simulink model "SpectrumAnalyzerMeasurements"  (R2024a)
settings: Solver=FixedStepDiscrete  StartTime=0.0  StopTime=100  RelTol=1e-3  EnableMultiTasking=on
libraries: dspsrcs4 x10, dsppolyfun x4, dspmlti4 x1
settings Model: Creator=The MathWorks, Inc.  LastModifiedBy=The MathWorks, Inc.
settings SolverCC: AlgebraicLoopSolver=TrustRegion  MaxZcPerStep=1
settings DataIOCC: LimitDataPoints=on  SaveFormat=Array  ReturnWorkspaceOutputs=off
settings OptimizationCC: LifeSpan=inf  SimCompilerOptimization=on
settings DebuggingCC: SolverPrmCheckMsg=warning  UnconnectedInputMsg=warning  UnconnectedOutputMsg=warning  UnconnectedLineMsg=warning  AllowSymbolicDim=off  SymbolicDimsDataTypeCodeGenerationDiagnostic=none  SFUnexpectedBacktrackingDiag=warning  SFNoUnconditionalDefaultTransitionDiag=warning  SFExecutionAtInitializationDiag=none  ArithmeticOperatorsInVariantConditions=warning
settings HardwareCC: ProdBitPerPointer=32  ProdBitPerSizeT=32  ProdBitPerPtrDiffT=32  ProdLargestAtomicFloat=None  ProdIntDivRoundTo=Undefined  ProdEndianess=Unspecified  ProdWordSize=32  ProdHWDeviceType=32-bit Generic
settings ModelReferenceCC: EnableRefExpFcnMdlSchedulingChecks=on  PropagateSignalLabelsOutOfModel=off
settings SFSimCC: SimUseLocalCustomCode=off  SimGenImportedTypeDefs=on  CustomCodeUndefinedFunction=UseInterfaceOnly
settings RTWCC: RTWUseLocalCustomCode=off  GPUComputeCapability=3.5  DLArmComputeVersion=19.05
settings CodeAppCC: StateflowObjectComments=on
settings GRTTargetCC: TargetLangStandard=C89/C90 (ANSI)
settings ConfigComp: CovMetricSettings=dw  CovSaveCumulativeToWorkspaceVar=on  CovSaveSingleToWorkspaceVar=on  CovExternalEMLEnable=off  CovSFcnEnable=off

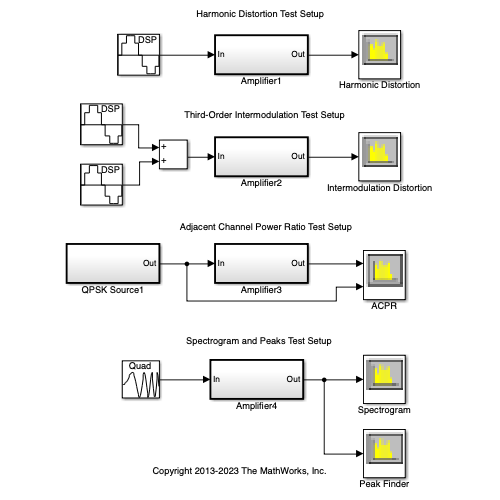
[thumbnail: Simulink's stored preview of the top-level diagram]
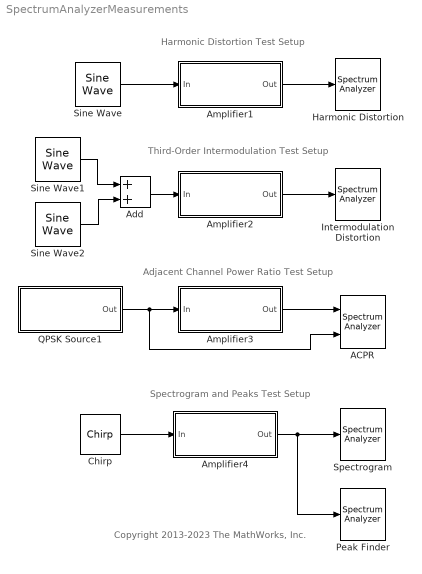
== system SpectrumAnalyzerMeasurements ==
  note: Spectrogram and Peaks Test Setup
  note: Adjacent Channel Power Ratio Test Setup
  note: Third-Order Intermodulation Test Setup
  note: Harmonic Distortion Test Setup
  note: Copyright 2013-2023 The MathWorks, Inc.
  ACPR : SpectrumAnalyzer  NumInputPorts=2  WindowPosition=[162.000000,32.000000,534.000000,420.000000,]  ScopeFrameLocation=window  Method=Welch  SampleRate=38400000  Span=1  StartFrequency=-0.5  StopFrequency=0.5  AveragingMethod=Running  YLabel=dBm  YLimits=[-119.21723774,40.57878414]  ShowLegend=on  AllowFFTLengthLessThanSamplesPerUpdate=on
  Add : Sum
  Amplifier1 : Subsystem  TreatAsAtomicUnit=on
  Amplifier2 : Subsystem  TreatAsAtomicUnit=on
  Amplifier3 : Subsystem  TreatAsAtomicUnit=on
  Amplifier4 : Subsystem  TreatAsAtomicUnit=on
  Chirp : dspsrcs4/Chirp  sweep=Quadratic  mode=Bidirectional  f0=2.5e6  f1=5e6  t1=1e-3  Tsweep=1e-3  phase=0  Ts=1/10/3.84e6  spf=10  datatype=double  OutputFrames=off
  Harmonic Distortion : SpectrumAnalyzer  WindowPosition=[109.000000,45.000000,549.000000,470.000000,]  ScopeFrameLocation=window  Method=Welch  SampleRate=38400000  PlotAsTwoSidedSpectrum=off  RBW=200e3  Span=500  CenterFrequency=250  StartFrequency=0  StopFrequency=500  Window=Kaiser  SidelobeAttenuation=190  OverlapPercent=80  AveragingMethod=Running  YLabel=dBm  YLimits=[-219.95441853,53.99786682]  SelectedToolstripTab=spectrumAnalyzerToolstrip.measurementsTab  AllowFFTLengthLessThanSamplesPerUpdate=on
  Intermodulation Distortion : SpectrumAnalyzer  WindowPosition=[136.000000,50.000000,548.000000,434.000000,]  ScopeFrameLocation=window  Method=Welch  SampleRate=38400000  PlotAsTwoSidedSpectrum=off  RBW=200e3  Span=500  CenterFrequency=250  StartFrequency=0  StopFrequency=500  Window=Kaiser  SidelobeAttenuation=190  OverlapPercent=80  AveragingMethod=Running  YLabel=dBm  YLimits=[-192.78808533,51.40291241]  SelectedToolstripTab=spectrumAnalyzerToolstrip.measurementsTab  AllowFFTLengthLessThanSamplesPerUpdate=on
  Peak Finder : SpectrumAnalyzer  WindowPosition=[229.000000,-33.000000,543.000000,420.000000,]  ScopeFrameLocation=window  Method=Welch  SampleRate=38400000  PlotAsTwoSidedSpectrum=off  AxesScaling=Manual  RBW=200e3  Span=1  StartFrequency=-0.5  StopFrequency=0.5  Window=Kaiser  SidelobeAttenuation=190  OverlapPercent=80  AveragingMethod=Running  YLabel=dBm  YLimits=[-199.63800241620794 51.208034885170299]  ColorLimits=[-250 1]  SelectedToolstripTab=spectrumAnalyzerToolstrip.measurementsTab  AllowFFTLengthLessThanSamplesPerUpdate=on
  QPSK Source1 : Subsystem  TreatAsAtomicUnit=on
  Sine Wave : dspsrcs4/Sine Wave  Amplitude=1  Frequency=2e6  Phase=0  SampleMode=Discrete  OutComplex=Real  CompMethod=Trigonometric fcn  TableSize=Speed  SampleTime=1/10/3.84e6  SamplesPerFrame=10  ResetState=Restart at time zero  OutputFrames=off  dataType=double  wordLen=16  udDataType=sfix(16)  fracBitsMode=Best precision  numFracBits=15  OutDataTypeStr=double  LastOutDataTypeStr=double
  Sine Wave1 : dspsrcs4/Sine Wave  Amplitude=1  Frequency=9e6  Phase=0  SampleMode=Discrete  OutComplex=Real  CompMethod=Trigonometric fcn  TableSize=Speed  SampleTime=1/10/3.84e6  SamplesPerFrame=10  ResetState=Restart at time zero  OutputFrames=off  dataType=double  wordLen=16  udDataType=sfix(16)  fracBitsMode=Best precision  numFracBits=15  OutDataTypeStr=double  LastOutDataTypeStr=double
  Sine Wave2 : dspsrcs4/Sine Wave  Amplitude=1  Frequency=11e6  Phase=0  SampleMode=Discrete  OutComplex=Real  CompMethod=Trigonometric fcn  TableSize=Speed  SampleTime=1/10/3.84e6  SamplesPerFrame=10  ResetState=Restart at time zero  OutputFrames=off  dataType=double  wordLen=16  udDataType=sfix(16)  fracBitsMode=Best precision  numFracBits=15  OutDataTypeStr=double  LastOutDataTypeStr=double
  Spectrogram : SpectrumAnalyzer  WindowPosition=[188.000000,0.000000,546.000000,420.000000,]  ScopeFrameLocation=window  ViewType=Spectrogram  Method=Welch  SampleRate=38400000  PlotAsTwoSidedSpectrum=off  AxesScaling=Manual  RBW=200e3  Span=1  StartFrequency=-0.5  StopFrequency=0.5  AveragingMethod=Running  TimeSpan=3e-3  YLabel="Time History (s)  \\rightarrow"  YLimits=[-111.46675674987713 39.602471793491674]  ColorLimits=[-150 20]  SelectedToolstripTab=spectrumAnalyzerToolstrip.measurementsTab  AllowFFTLengthLessThanSamplesPerUpdate=on
  wires:
  Amplifier1/1(Out) -> Harmonic Distortion/1
  Sine Wave/1 -> Amplifier1/1(In)
  Sine Wave1/1 -> Add/1
  Sine Wave2/1 -> Add/2
  Add/1 -> Amplifier2/1(In)
  Amplifier2/1(Out) -> Intermodulation Distortion/1
  QPSK Source1/1(Out) -> ACPR/2, Amplifier3/1(In)
  Amplifier3/1(Out) -> ACPR/1
  Chirp/1 -> Amplifier4/1(In)
  Amplifier4/1(Out) -> Peak Finder/1, Spectrogram/1

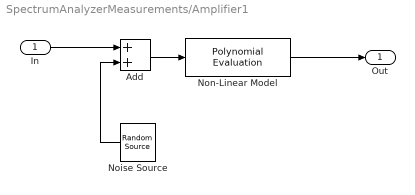
== system SpectrumAnalyzerMeasurements/Amplifier1 ==
  In : Inport
  Add : Sum
  Noise Source : dspsrcs4/Random Source  SrcType=Gaussian  MinVal=0  MaxVal=1  MeanVal=0  VarVal=4e-16  RepMode=Not repeatable  rawSeed=1  IsInherit=off  SampTime=1/10/3.84e6  SampFrame=10  OutComplex=Real  DataType=double  SimulateUsing=Interpreted execution
  Non-Linear Model : dsppolyfun/Polynomial Evaluation  useConstCoeffs=on  constCoeffs=[1e-6 1e-9 1e-5 1e-9 1e-6 5e-8 .5e-3 1e-6 1 3e-3]
  Out : Outport  VectorParamsAs1DForOutWhenUnconnected=off
  wires:
  Non-Linear Model/1 -> Out/1
  In/1 -> Add/1
  Add/1 -> Non-Linear Model/1
  Noise Source/1 -> Add/2

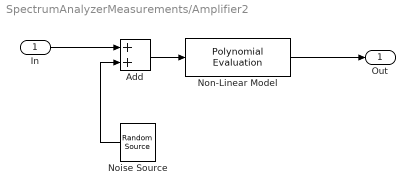
== system SpectrumAnalyzerMeasurements/Amplifier2 ==
  In : Inport
  Add : Sum
  Noise Source : dspsrcs4/Random Source  SrcType=Gaussian  MinVal=0  MaxVal=1  MeanVal=0  VarVal=4e-14  RepMode=Not repeatable  rawSeed=1  IsInherit=off  SampTime=1/10/3.84e6  SampFrame=10  OutComplex=Real  DataType=double  SimulateUsing=Interpreted execution
  Non-Linear Model : dsppolyfun/Polynomial Evaluation  useConstCoeffs=on  constCoeffs=[1e-6 1e-9 1e-5 1e-9 1e-6 5e-8 .5e-3 1e-6 1 3e-3]
  Out : Outport  VectorParamsAs1DForOutWhenUnconnected=off
  wires:
  Non-Linear Model/1 -> Out/1
  In/1 -> Add/1
  Add/1 -> Non-Linear Model/1
  Noise Source/1 -> Add/2

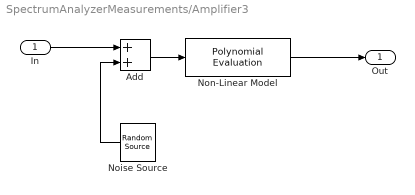
== system SpectrumAnalyzerMeasurements/Amplifier3 ==
  In : Inport
  Add : Sum
  Noise Source : dspsrcs4/Random Source  SrcType=Gaussian  MinVal=0  MaxVal=1  MeanVal=0  VarVal=4e-14  RepMode=Not repeatable  rawSeed=1  IsInherit=off  SampTime=1/10/3.84e6  SampFrame=10  OutComplex=Real  DataType=double  SimulateUsing=Interpreted execution
  Non-Linear Model : dsppolyfun/Polynomial Evaluation  useConstCoeffs=on  constCoeffs=[1e-6 1e-9 1e-5 1e-9 1e-6 5e-8 .5e-3 1e-6 1 3e-3]
  Out : Outport  VectorParamsAs1DForOutWhenUnconnected=off
  wires:
  Non-Linear Model/1 -> Out/1
  In/1 -> Add/1
  Add/1 -> Non-Linear Model/1
  Noise Source/1 -> Add/2

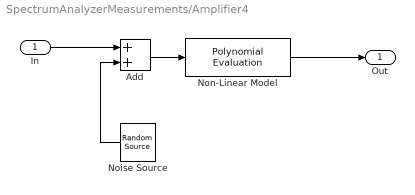
== system SpectrumAnalyzerMeasurements/Amplifier4 ==
  In : Inport
  Add : Sum
  Noise Source : dspsrcs4/Random Source  SrcType=Gaussian  MinVal=0  MaxVal=1  MeanVal=0  VarVal=4e-14  RepMode=Not repeatable  rawSeed=1  IsInherit=off  SampTime=1/10/3.84e6  SampFrame=10  OutComplex=Real  DataType=double  SimulateUsing=Interpreted execution
  Non-Linear Model : dsppolyfun/Polynomial Evaluation  useConstCoeffs=on  constCoeffs=[1e-6 1e-9 1e-5 1e-9 1e-6 5e-8 .5e-3 1e-6 1 3e-3]
  Out : Outport  VectorParamsAs1DForOutWhenUnconnected=off
  wires:
  Non-Linear Model/1 -> Out/1
  In/1 -> Add/1
  Add/1 -> Non-Linear Model/1
  Noise Source/1 -> Add/2

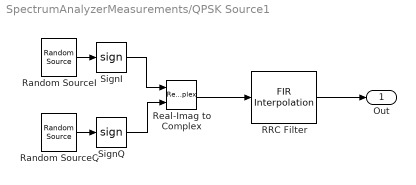
== system SpectrumAnalyzerMeasurements/QPSK Source1 ==
  RRC Filter : dspmlti4/FIR Interpolation  FilterSource=Dialog parameters  PrivateCoeffs=0  h=5*rcosdesign(0.5, 20, 10, 'sqrt')  L=10  FilterObject=Hm_firinterp  InputProcessing=Columns as channels (frame based)  framing=Enforce single-rate processing  outputBufInitCond=0  roundingMode=Floor  overflowMode=off  firstCoeffDataTypeStr=Inherit: Same word length as input  firstCoeffMin=[]  firstCoeffMax=[]  firstCoeffLastDataTypeStr=Inherit: Same word length as input  outputDataTypeStr=Inherit: Same as accumulator  outputMin=[]  outputMax=[]  outputLastDataTypeStr=Inherit: Same as accumulator
  Random SourceI : dspsrcs4/Random Source  SrcType=Uniform  MinVal=-1  MaxVal=1  MeanVal=0  VarVal=1  RepMode=Not repeatable  rawSeed=1  IsInherit=off  SampTime=1/3.84e6  SampFrame=1  OutComplex=Real  DataType=double  SimulateUsing=Interpreted execution
  Random SourceQ : dspsrcs4/Random Source  SrcType=Uniform  MinVal=-1  MaxVal=1  MeanVal=0  VarVal=1  RepMode=Not repeatable  rawSeed=1  IsInherit=off  SampTime=1/3.84e6  SampFrame=1  OutComplex=Real  DataType=double  SimulateUsing=Interpreted execution
  Real-Imag to Complex : RealImagToComplex
  SignI : Signum
  SignQ : Signum
  Out : Outport  VectorParamsAs1DForOutWhenUnconnected=off
  wires:
  Random SourceI/1 -> SignI/1
  Random SourceQ/1 -> SignQ/1
  SignI/1 -> Real-Imag to Complex/1
  SignQ/1 -> Real-Imag to Complex/2
  Real-Imag to Complex/1 -> RRC Filter/1
  RRC Filter/1 -> Out/1
